simulink library "aero_drag_lib"  (R2016b)
settings: Solver=VariableStepAuto  StartTime=0.0  StopTime=10.0  RelTol=1e-3
undefined symbols (not defined in the file or in its folder): Earth, sim_params, WGS84
libraries: aerolibtransform2 x1, aerolibatmos2 x1, aerolibutil x1
settings Model: Creator=bbarz_000  LastModifiedBy=taylorreynolds
settings OptimizationCC: LifeSpan=inf
settings DebuggingCC: SFExecutionAtInitializationDiag=none

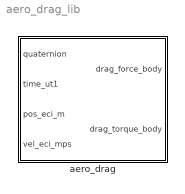
== system aero_drag_lib ==
  aero_drag : Subsystem

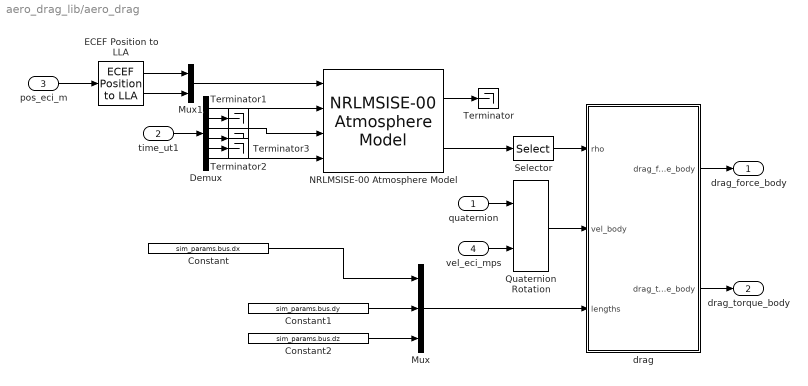
== system aero_drag_lib/aero_drag ==
  quaternion : Inport
  time_ut1 : Inport  Port=2
  pos_eci_m : Inport  Port=3
  vel_eci_mps : Inport  Port=4
  Constant : Constant  Value=sim_params.bus.dx
  Constant1 : Constant  Value=sim_params.bus.dy
  Constant2 : Constant  Value=sim_params.bus.dz
  Demux : Demux  Outputs=6
  ECEF Position to LLA : aerolibtransform2/ECEF Position to LLA  units=Metric (MKS)  ptype=Earth (WGS84)  F=1/298.257223563  R=6378137
  Mux : Mux  Inputs=3
  Mux1 : Mux  Inputs=2
  NRLMSISE-00 Atmosphere Model : aerolibatmos2/NRLMSISE-00 Atmosphere Model  units=Metric (MKS)  lst_input=off  flux_ap_input=off  flags_input=Internal  flags=ones(1,23)  oxygen_in=off  action=Warning
  Quaternion Rotation : aerolibutil/Quaternion Rotation
  Selector : Selector  InputPortWidth=9  IndexOptions=Index vector (dialog)  Indices=6  OutputSizes=1
  Terminator{,1..3} (4 alike) : Terminator
  drag : MATLAB Function  TreatAsAtomicUnit=on
  drag_force_body : Outport
  drag_torque_body : Outport  Port=2
  wires:
  quaternion/1 -> Quaternion Rotation/1
  vel_eci_mps/1 -> Quaternion Rotation/2
  drag/1(drag_force_body) -> drag_force_body/1
  drag/2(drag_torque_body) -> drag_torque_body/1
  Quaternion Rotation/1 -> drag/2(vel_body)
  Constant/1 -> Mux/1
  Constant1/1 -> Mux/2
  Constant2/1 -> Mux/3
  Mux/1 -> drag/3(lengths)
  Selector/1 -> drag/1(rho)
  NRLMSISE-00 Atmosphere Model/2 -> Selector/1
  NRLMSISE-00 Atmosphere Model/1 -> Terminator/1
  time_ut1/1 -> Demux/1
  Demux/6 -> NRLMSISE-00 Atmosphere Model/4
  Demux/3 -> NRLMSISE-00 Atmosphere Model/3
  Demux/1 -> NRLMSISE-00 Atmosphere Model/2
  Demux/2 -> Terminator1/1
  Demux/4 -> Terminator2/1
  Demux/5 -> Terminator3/1
  pos_eci_m/1 -> ECEF Position to LLA/1
  Mux1/1 -> NRLMSISE-00 Atmosphere Model/1
  ECEF Position to LLA/2 -> Mux1/2
  ECEF Position to LLA/1 -> Mux1/1

== matlab function aero_drag_lib/aero_drag/drag ==
  data: drag_force_body output size=3; drag_torque_body output size=3; rho input; vel_body input; lengths input
function [drag_force_body, drag_torque_body] = drag_force(rho, vel_body, lengths)
%#codegen

lenx    = lengths(1);
leny    = lengths(2);
lenz    = lengths(3);
% q       = sc_quat;
% DCM     = my_quat2dcm(q);
% center_of_mass = reshape(COM, [3 1]);
vel_body = reshape(vel_body, [3 1]);

vel_unit = vel_body/norm(vel_body);

%c = 2.5; % Drag coefficient..do we need this?

% Define std body vectors in body frame
body_vecs = [1 0 0;
            -1 0 0;
            0 1 0;
            0 -1 0;
            0 0 1;
            0 0 -1]';
        
% Rotate body vectors to account for current orientation
% rot_body_vecs   = DCM*body_vecs;       

centroid_vecs = [0.05 0 0;
                -0.05 0 0;
                0 0.05 0;
                0 -0.05 0;
                0 0 0.15;
                0 0 -0.15]'; %- center_of_mass*ones(1,6);

% Compute areas for each face
areas   = [leny*lenz,leny*lenz,lenx*lenz,lenx*lenz,lenx*leny,lenx*leny];

dot_prod = zeros(1,6);
f = zeros(3,6);
cop = zeros(3,6);

for i = 1:6
    if dot(vel_body, body_vecs(:,i)) > 0
        dot_prod(i) = dot(body_vecs(:,i),vel_unit);
        f(:,i) = -rho*norm(vel_body)^2*areas(i)*dot_prod(i)*vel_unit;
        cop(:,i) = centroid_vecs(:,i)*dot_prod(i);
%        tau(:,i) = cross(centroid_vecs(:,i), f(:,i));
    end
end
center_pressure_body = sum(cop, 2)/sum(dot_prod, 2);
drag_force_body = sum(f, 2);
drag_torque_body = cross(center_pressure_body, drag_force_body);

end
